simulink model "simulinkanwser"  (R2021a)
settings: Solver=VariableStepAuto  StartTime=0.0  StopTime=100  RelTol=1e-3  AbsTol=1e-3
settings Model: Creator=huangzijing  LastModifiedBy=huangzijing
settings SolverCC: AutoScaleAbsTol=off  AlgebraicLoopSolver=TrustRegion
settings DebuggingCC: SymbolicDimsDataTypeCodeGenerationDiagnostic=none  SFMachineParentedDataDiag=warning
settings SFSimCC: CustomCodeUndefinedFunction=UseInterfaceOnly
settings SimscapeCC: SimscapeLogType=all  SimscapeLogSimulationStatistics=on  SimscapeLogDataHistory=10000

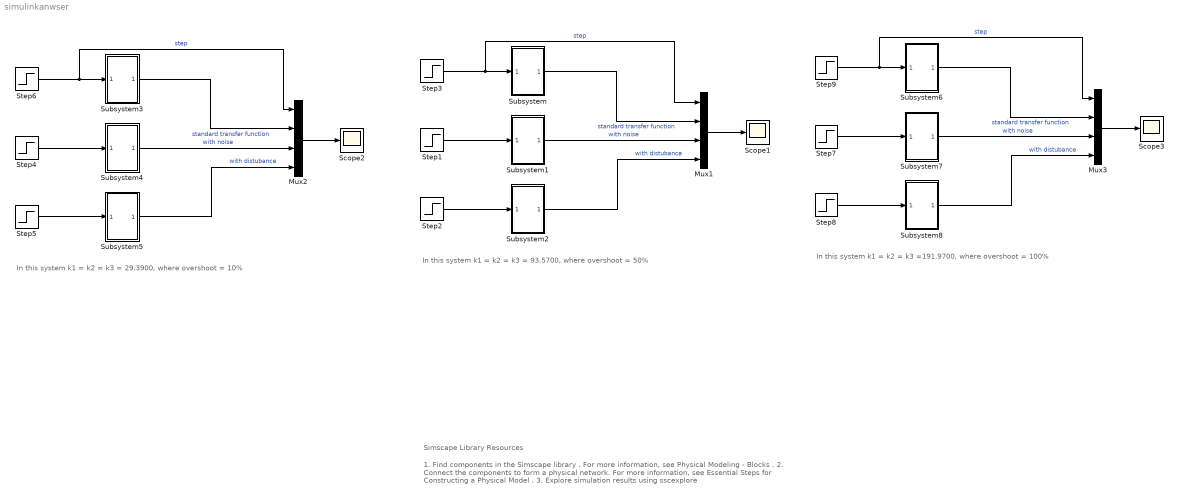
== system simulinkanwser ==
  note: 1. Find components in the Simscape library .
      | For more information, see Physical Modeling - Blocks .
      | 2. Connect the components to form a physical network.
      | For more information, see Essential Steps for Constructing a Physical Model .
      | 3. Explore simulation results using sscexplore
  note: Simscape Library Resources
  note: In this system k1 = k2 = k3 = 93.5700, where overshoot = 50%
  note: In this system k1 = k2 = k3 = 29.3900, where overshoot = 10%
  note: In this system k1 = k2 = k3 =191.9700, where overshoot = 100%
  Mux1 : Mux
  Mux2 : Mux
  Mux3 : Mux
  Scope1 : Scope
  Scope2 : Scope
  Scope3 : Scope
  Step{1..9} (9 alike) : Step  SampleTime=0
  Subsystem : Subsystem
  Subsystem1 : Subsystem
  Subsystem2 : Subsystem
  Subsystem3 : Subsystem
  Subsystem4 : Subsystem
  Subsystem5 : Subsystem
  Subsystem6 : Subsystem
  Subsystem7 : Subsystem
  Subsystem8 : Subsystem
  wires:
  Mux1/1 -> Scope1/1
  Step3/1 -> Mux1/1, Subsystem/1(In1)  "step"
  Subsystem/1(Out1) -> Mux1/2  "standard transfer function"
  Step1/1 -> Subsystem1/1(In1)
  Subsystem1/1(Out1) -> Mux1/3  "with noise"
  Step2/1 -> Subsystem2/1(In1)
  Subsystem2/1(Out1) -> Mux1/4  "with distubance"
  Subsystem5/1(Out1) -> Mux2/4  "with distubance"
  Step4/1 -> Subsystem4/1(In1)
  Step6/1 -> Mux2/1, Subsystem3/1(In1)  "step"
  Subsystem4/1(Out1) -> Mux2/3  "with noise"
  Subsystem3/1(Out1) -> Mux2/2  "standard transfer function"
  Step5/1 -> Subsystem5/1(In1)
  Mux2/1 -> Scope2/1
  Step9/1 -> Mux3/1, Subsystem6/1(In1)  "step"
  Step7/1 -> Subsystem7/1(In1)
  Subsystem7/1(Out1) -> Mux3/3  "with noise"
  Subsystem6/1(Out1) -> Mux3/2  "standard transfer function"
  Subsystem8/1(Out1) -> Mux3/4  "with distubance"
  Step8/1 -> Subsystem8/1(In1)
  Mux3/1 -> Scope3/1

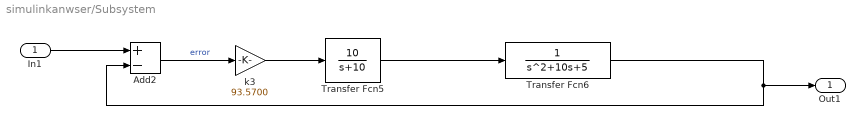
== system simulinkanwser/Subsystem ==
  In1 : Inport
  Add2 : Sum  Inputs=+-
  Transfer Fcn5 : TransferFcn  Numerator=[10]  Denominator=[1 10]
  Transfer Fcn6 : TransferFcn  Denominator=[1 10 5]
  k3 : Gain  Gain=93.5700
  Out1 : Outport
  wires:
  In1/1 -> Add2/1
  Transfer Fcn6/1 -> Add2/2, Out1/1
  Transfer Fcn5/1 -> Transfer Fcn6/1
  Add2/1 -> k3/1  "error"
  k3/1 -> Transfer Fcn5/1

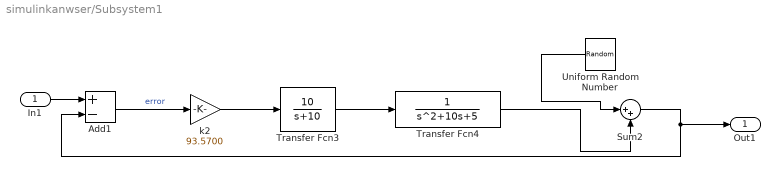
== system simulinkanwser/Subsystem1 ==
  In1 : Inport
  Add1 : Sum  Inputs=+-
  Sum2 : Sum  Inputs=|++
  Transfer Fcn3 : TransferFcn  Numerator=[10]  Denominator=[1 10]
  Transfer Fcn4 : TransferFcn  Denominator=[1 10 5]
  Uniform Random Number : UniformRandomNumber  Minimum=-0.1  Maximum=0.1  SampleTime=0.1
  k2 : Gain  Gain=93.5700
  Out1 : Outport
  wires:
  Transfer Fcn3/1 -> Transfer Fcn4/1
  k2/1 -> Transfer Fcn3/1
  Add1/1 -> k2/1  "error"
  In1/1 -> Add1/1
  Sum2/1 -> Add1/2, Out1/1
  Uniform Random Number/1 -> Sum2/1
  Transfer Fcn4/1 -> Sum2/2

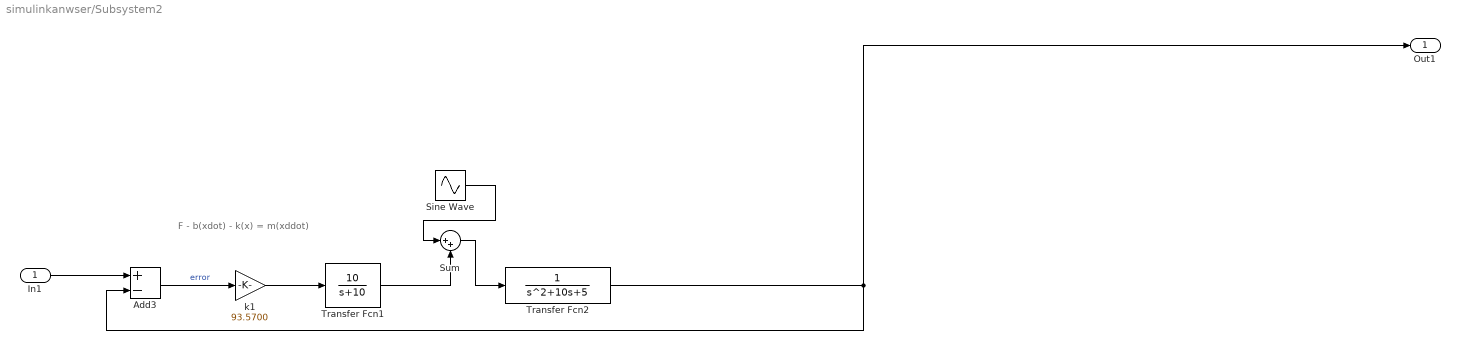
== system simulinkanwser/Subsystem2 ==
  note: F - b(xdot) - k(x) = m(xddot)
  In1 : Inport
  Add3 : Sum  Inputs=+-
  Sine Wave : Sin  Amplitude=0.5  SampleTime=0
  Sum : Sum  Inputs=|++
  Transfer Fcn1 : TransferFcn  Numerator=[10]  Denominator=[1 10]
  Transfer Fcn2 : TransferFcn  Denominator=[1 10 5]
  k1 : Gain  Gain=93.5700
  Out1 : Outport
  wires:
  In1/1 -> Add3/1
  Transfer Fcn1/1 -> Sum/2
  Transfer Fcn2/1 -> Out1/1, Add3/2
  k1/1 -> Transfer Fcn1/1
  Sum/1 -> Transfer Fcn2/1
  Add3/1 -> k1/1  "error"
  Sine Wave/1 -> Sum/1

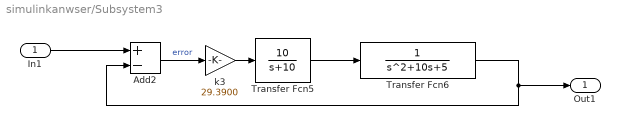
== system simulinkanwser/Subsystem3 ==
  In1 : Inport
  Add2 : Sum  Inputs=+-
  Transfer Fcn5 : TransferFcn  Numerator=[10]  Denominator=[1 10]
  Transfer Fcn6 : TransferFcn  Denominator=[1 10 5]
  k3 : Gain  Gain=29.3900
  Out1 : Outport
  wires:
  In1/1 -> Add2/1
  Transfer Fcn6/1 -> Add2/2, Out1/1
  Transfer Fcn5/1 -> Transfer Fcn6/1
  Add2/1 -> k3/1  "error"
  k3/1 -> Transfer Fcn5/1

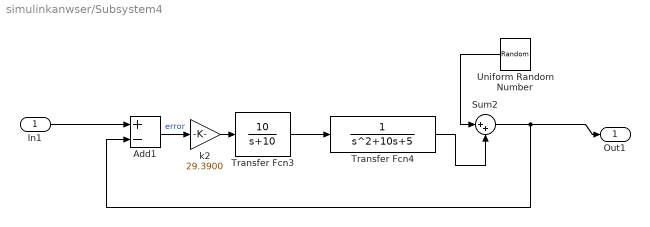
== system simulinkanwser/Subsystem4 ==
  In1 : Inport
  Add1 : Sum  Inputs=+-
  Sum2 : Sum  Inputs=|++
  Transfer Fcn3 : TransferFcn  Numerator=[10]  Denominator=[1 10]
  Transfer Fcn4 : TransferFcn  Denominator=[1 10 5]
  Uniform Random Number : UniformRandomNumber  Minimum=-0.1  Maximum=0.1  SampleTime=0.1
  k2 : Gain  Gain=29.3900
  Out1 : Outport
  wires:
  Transfer Fcn3/1 -> Transfer Fcn4/1
  k2/1 -> Transfer Fcn3/1
  Add1/1 -> k2/1  "error"
  In1/1 -> Add1/1
  Uniform Random Number/1 -> Sum2/1
  Transfer Fcn4/1 -> Sum2/2
  Sum2/1 -> Out1/1, Add1/2

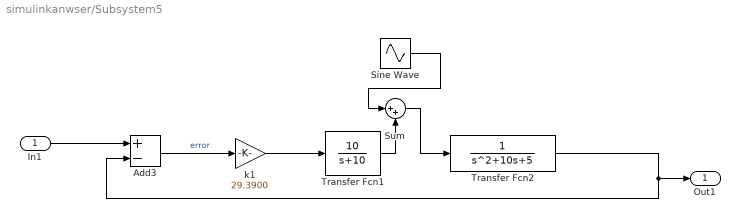
== system simulinkanwser/Subsystem5 ==
  In1 : Inport
  Add3 : Sum  Inputs=+-
  Sine Wave : Sin  Amplitude=0.5  SampleTime=0
  Sum : Sum  Inputs=|++
  Transfer Fcn1 : TransferFcn  Numerator=[10]  Denominator=[1 10]
  Transfer Fcn2 : TransferFcn  Denominator=[1 10 5]
  k1 : Gain  Gain=29.3900
  Out1 : Outport
  wires:
  In1/1 -> Add3/1
  Transfer Fcn1/1 -> Sum/2
  Transfer Fcn2/1 -> Out1/1, Add3/2
  k1/1 -> Transfer Fcn1/1
  Sum/1 -> Transfer Fcn2/1
  Add3/1 -> k1/1  "error"
  Sine Wave/1 -> Sum/1

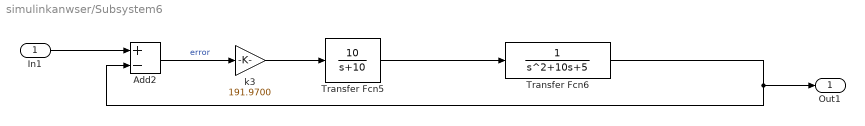
== system simulinkanwser/Subsystem6 ==
  In1 : Inport
  Add2 : Sum  Inputs=+-
  Transfer Fcn5 : TransferFcn  Numerator=[10]  Denominator=[1 10]
  Transfer Fcn6 : TransferFcn  Denominator=[1 10 5]
  k3 : Gain  Gain=191.9700
  Out1 : Outport
  wires:
  In1/1 -> Add2/1
  Transfer Fcn6/1 -> Add2/2, Out1/1
  Transfer Fcn5/1 -> Transfer Fcn6/1
  Add2/1 -> k3/1  "error"
  k3/1 -> Transfer Fcn5/1

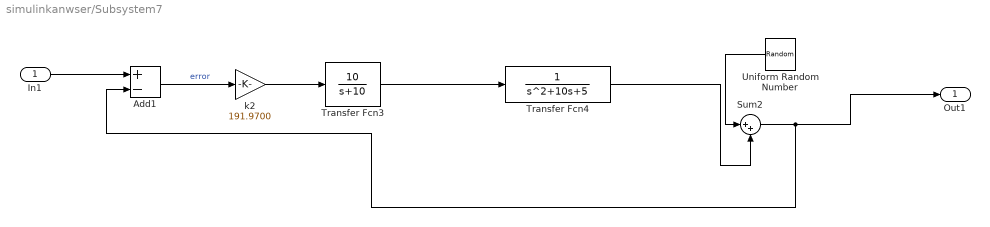
== system simulinkanwser/Subsystem7 ==
  In1 : Inport
  Add1 : Sum  Inputs=+-
  Sum2 : Sum  Inputs=|++
  Transfer Fcn3 : TransferFcn  Numerator=[10]  Denominator=[1 10]
  Transfer Fcn4 : TransferFcn  Denominator=[1 10 5]
  Uniform Random Number : UniformRandomNumber  Minimum=-0.1  Maximum=0.1  SampleTime=0.1
  k2 : Gain  Gain=191.9700
  Out1 : Outport
  wires:
  Transfer Fcn3/1 -> Transfer Fcn4/1
  k2/1 -> Transfer Fcn3/1
  Add1/1 -> k2/1  "error"
  In1/1 -> Add1/1
  Sum2/1 -> Add1/2, Out1/1
  Uniform Random Number/1 -> Sum2/1
  Transfer Fcn4/1 -> Sum2/2

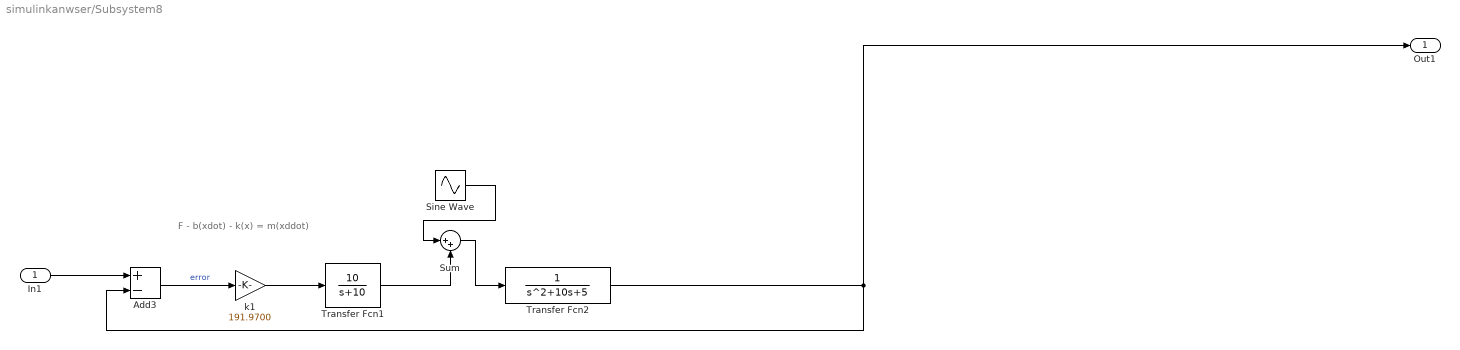
== system simulinkanwser/Subsystem8 ==
  note: F - b(xdot) - k(x) = m(xddot)
  In1 : Inport
  Add3 : Sum  Inputs=+-
  Sine Wave : Sin  Amplitude=0.5  SampleTime=0
  Sum : Sum  Inputs=|++
  Transfer Fcn1 : TransferFcn  Numerator=[10]  Denominator=[1 10]
  Transfer Fcn2 : TransferFcn  Denominator=[1 10 5]
  k1 : Gain  Gain=191.9700
  Out1 : Outport
  wires:
  In1/1 -> Add3/1
  Transfer Fcn1/1 -> Sum/2
  Transfer Fcn2/1 -> Out1/1, Add3/2
  k1/1 -> Transfer Fcn1/1
  Sum/1 -> Transfer Fcn2/1
  Add3/1 -> k1/1  "error"
  Sine Wave/1 -> Sum/1
